simulink model "Progetto_Gruppo21_IZ"  (R2024b)
settings: Solver=FixedStepDiscrete  StartTime=0.0  StopTime=300  FixedStep=0.5  RelTol=1e-3  EnableMultiTasking=on
libraries: stm32f4xxblockslib x6, stm32g4xxblockslib x2, stm32blockslib x2
settings Model: STM32="{\"UARTRead\":{\"ID\":\"Progetto_Gruppo21_IZ:67\"},\"UARTWrite\":{\"ID\":\"Progetto_Gruppo21_IZ:69\"},\"DigitalPortRead\":[{\"ID\":\"Progetto_Gruppo21_IZ:71\"},{\"ID\":\"Progetto_Gruppo21_IZ:72\"},{\"ID\":\"Progetto_Gruppo21_IZ:73\"},{\"ID\":\"Progetto_Gruppo21_IZ:74\"}],\"DigitalPortWrite\":[{\"ID\":\"Progetto_Gruppo21_IZ:75\"},{\"ID\":\"Progetto_Gruppo21_IZ:76\"}],\"PWMOutput\":[{\"ID\":\"Progetto_Gruppo21_IZ:78\"},{\"ID\":\"Progetto_Gruppo21_IZ:80\"}]}"  PacingRate=0.500000  Creator=angel  LastModifiedBy=angel
settings OptimizationCC: DefaultParameterBehavior=Inlined  EnhancedBackFolding=on  PassReuseOutputArgsAs=Individual arguments  ZeroExternalMemoryAtStartup=off  ZeroInternalMemoryAtStartup=off  MaxStackSize=512  OptimizeBlockOrder=speed  DifferentSizesBufferReuse=on  OptimizationCustomize=off  EfficientTunableParamExpr=on
settings DebuggingCC: ParameterTunabilityLossMsg=error
settings HardwareCC: ProdBitPerPointer=32  ProdBitPerSizeT=32  ProdBitPerPtrDiffT=32  ProdLargestAtomicInteger=Long  ProdLargestAtomicFloat=Double  ProdWordSize=32  ProdLongLongMode=on  ProdHWDeviceType=ARM Compatible->ARM Cortex-M
settings RTWCC: Description=Embedded Coder  SystemTargetFile=ert.tlc  HardwareBoard=STM32G4xx Based  TemplateMakefile=ert_default_tmf  Toolchain=GNU Tools for ARM Embedded Processors
settings CodeAppCC: ForceParamTrailComments=on  IgnoreCustomStorageClasses=off  OperatorAnnotations=on  SimulinkDataObjDesc=on  SFDataObjDesc=on  InsertBlockDesc=on
settings ERTTargetCC: TargetLangStandard=C99 (ISO)  CodeReplacementLibrary=ARM Cortex-M  SupportVariableSizeSignals=on  ExtModeTransport=3  ExtModeStaticAlloc=on  ExtModeStaticAllocSize=2048  ExtModeMexFile=ext_xcp  ExtModeIntrfLevel=Level2 - Open

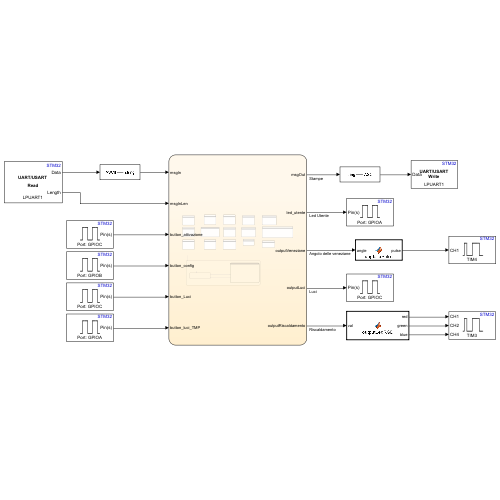
[thumbnail: Simulink's stored preview of the top-level diagram]
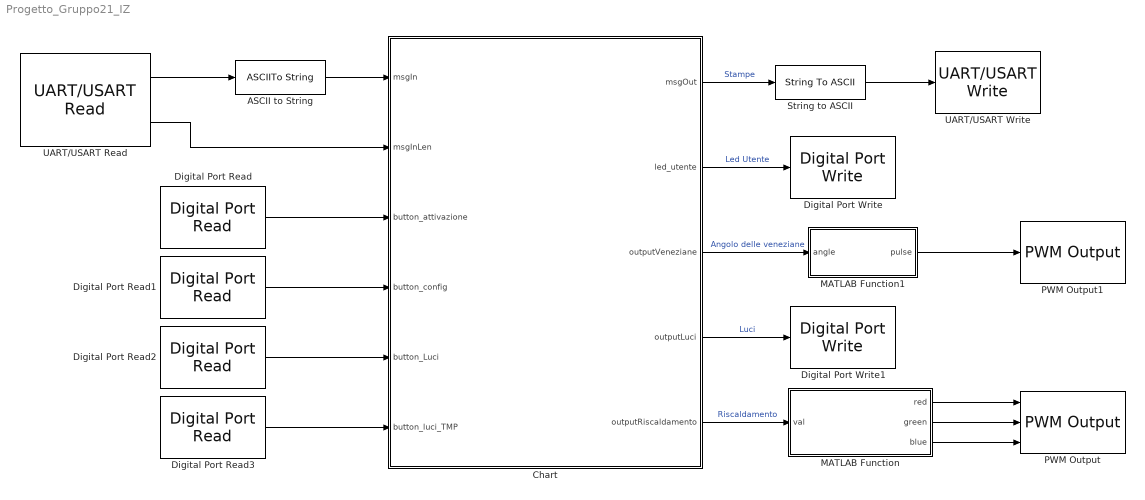
== system Progetto_Gruppo21_IZ ==
  ASCII to String : ASCIIToString
  Chart : Stateflow chart  TreatAsAtomicUnit=on
  Digital Port Read : stm32f4xxblockslib/Digital Port Read  PortName=GPIOC  PinNumber=[13]  ReadOperation=on  IOAsArray=on  SampleTime=-1  EnableSimPort=off  hoistedMaskSrc=ECSoC/ECSimCodegen/Digital Port Read
      settings: LibrarySourceBlock=stm32g4xxblockslib/Digital Port Read
  Digital Port Read1 : stm32f4xxblockslib/Digital Port Read  PortName=GPIOB  PinNumber=[0]  ReadOperation=on  IOAsArray=on  SampleTime=-1  EnableSimPort=off  hoistedMaskSrc=ECSoC/ECSimCodegen/Digital Port Read
      settings: LibrarySourceBlock=stm32g4xxblockslib/Digital Port Read
  Digital Port Read2 : stm32f4xxblockslib/Digital Port Read  PortName=GPIOC  PinNumber=[10]  ReadOperation=on  IOAsArray=on  SampleTime=-1  EnableSimPort=off  hoistedMaskSrc=ECSoC/ECSimCodegen/Digital Port Read
      settings: LibrarySourceBlock=stm32g4xxblockslib/Digital Port Read
  Digital Port Read3 : stm32f4xxblockslib/Digital Port Read  PortName=GPIOA  PinNumber=[15]  ReadOperation=on  IOAsArray=on  SampleTime=-1  EnableSimPort=off  hoistedMaskSrc=ECSoC/ECSimCodegen/Digital Port Read
      settings: LibrarySourceBlock=stm32g4xxblockslib/Digital Port Read
  Digital Port Write : stm32f4xxblockslib/Digital Port Write  PortName=GPIOA  PinNumber=[5]  ReadOperation=off  IOAsArray=on  EnableSimPort=off  hoistedMaskSrc=ECSoC/ECSimCodegen/Digital Port Write
      settings: LibrarySourceBlock=stm32g4xxblockslib/Digital Port Write
  Digital Port Write1 : stm32f4xxblockslib/Digital Port Write  PortName=GPIOC  PinNumber=[2]  ReadOperation=off  IOAsArray=on  EnableSimPort=off  hoistedMaskSrc=ECSoC/ECSimCodegen/Digital Port Write
      settings: LibrarySourceBlock=stm32g4xxblockslib/Digital Port Write
  MATLAB Function : MATLAB Function  TreatAsAtomicUnit=on
  MATLAB Function1 : MATLAB Function  TreatAsAtomicUnit=on
  PWM Output : stm32g4xxblockslib/PWM Output  TimerModule=TIM3  DutycycleUnits=Counts  EnableChannel1=on  EnableChannel2=on  EnableChannel3=off  EnableChannel4=on  EnableChannel5=off  EnableChannel6=off  EnableCounterInput=off  EnableMainOutputInput=off  EnableFrequencyInput=off  SetRCAfterCE=off  OutputDirection=off  OutputMainOutputEnableStatus=off  SampleTime=0.1  EnableSimPort=off  EnableUpdateEvent=off  EnableCaptureCompare1Event=off  EnableCaptureCompare2Event=off  EnableCaptureCompare3Event=off  EnableCaptureCompare4Event=off  EnableTriggerEvent=off  EnableBreakEvent=off  EnableBreakEvent2=off  ProcessorFamily=STM32G4  hoistedMaskSrc=ECSoC/ECSimCodegen/PWM Output
  PWM Output1 : stm32g4xxblockslib/PWM Output  TimerModule=TIM4  DutycycleUnits=Counts  EnableChannel1=on  EnableChannel2=off  EnableChannel3=off  EnableChannel4=off  EnableChannel5=off  EnableChannel6=off  EnableCounterInput=off  EnableMainOutputInput=off  EnableFrequencyInput=off  SetRCAfterCE=off  OutputDirection=off  OutputMainOutputEnableStatus=off  SampleTime=0.1  EnableSimPort=off  EnableUpdateEvent=off  EnableCaptureCompare1Event=off  EnableCaptureCompare2Event=off  EnableCaptureCompare3Event=off  EnableCaptureCompare4Event=off  EnableTriggerEvent=off  EnableBreakEvent=off  EnableBreakEvent2=off  ProcessorFamily=STM32G4  hoistedMaskSrc=ECSoC/ECSimCodegen/PWM Output
  String to ASCII : StringToASCII  OutputVectorSize=127
  UART/USART Read : stm32blockslib/UART//USART Read  UARTModule=LPUART1  DataType=uint8  DataLength=1  BlockingMode=off  BlockingTimeout=0.1  OutputLength=on  OutputStatus=off  SampleTime=-1
      settings: LibrarySourceBlock=stm32g4xxblockslib/UART//USART Read
  UART/USART Write : stm32blockslib/UART//USART Write  UARTModule=LPUART1  LengthOfDataToSend=off  BlockingMode=off  BlockingTimeout=0.1  OutputStatus=off
      settings: LibrarySourceBlock=stm32g4xxblockslib/UART//USART Write
  wires:
  ASCII to String/1 -> Chart/1(msgIn)
  UART/USART Read/1 -> ASCII to String/1
  UART/USART Read/2 -> Chart/2(msgInLen)
  Chart/1(msgOut) -> String to ASCII/1  "Stampe"
  String to ASCII/1 -> UART/USART Write/1
  Digital Port Read/1 -> Chart/3(button_attivazione)
  Digital Port Read1/1 -> Chart/4(button_config)
  Digital Port Read2/1 -> Chart/5(button_Luci)
  Digital Port Read3/1 -> Chart/6(button_luci_TMP)
  Chart/4(outputLuci) -> Digital Port Write1/1  "Luci"
  Chart/2(led_utente) -> Digital Port Write/1  "Led Utente"
  Chart/5(outputRiscaldamento) -> MATLAB Function/1(val)  "Riscaldamento"
  MATLAB Function/1(red) -> PWM Output/1
  MATLAB Function/2(green) -> PWM Output/2
  MATLAB Function/3(blue) -> PWM Output/3
  Chart/3(outputVeneziane) -> MATLAB Function1/1(angle)  "Angolo delle veneziane"
  MATLAB Function1/1(pulse) -> PWM Output1/1

== matlab function Progetto_Gruppo21_IZ/MATLAB Function1 ==
  data: angle input; pulse output
function pulse = angleToPulse(angle)
    pulse = ((angle/180)*2000) + 500;
end

== matlab function Progetto_Gruppo21_IZ/MATLAB Function ==
  data: val input; red output; green output; blue output
function [red,green,blue] = outputLedRGD(val)
    switch val
        case 0
            red = 0;
            green = 0;
            blue = 255;
        case 1
            red = 155;
            green = 0;
            blue = 155;
        case 2
            red = 255;
            green = 90;
            blue = 0;
        case 3
            red = 255;
            green = 20;
            blue = 0;
        case 4
            red = 255;
            green = 0;
            blue = 0;
        otherwise
            red = 0;
            green = 0;
            blue = 0;
end

== stateflow chart Progetto_Gruppo21_IZ/Chart ==
  state Inizializzazione
    state Stato_Attivo
      state Gestione_Pulsanti_Luci [parallel]
        settings: executionOrder=3
        state Stato_di_Attesa
        state Gestore_pulsante_Luci_TMP
          state Caso_luci_accese
            en: luci = 3;
            du:
            if luci ~= 3
            stopTimer = true;
            end
          state Caso_luci_spente
            en: luci = 3;
            outputLuci = ON;
            du:
            if luci ~= 3
            stopTimer = true;
            end
          state Fine_Tempo
            en: luci = 2;
            outputLuci = OFF;
          (default) -> (junction 807) : {stopTimer = false}
          (junction 807) -> Inizializzazione.Stato_Attivo.Gestione_Pulsanti_Luci.Gestore_pulsante_Luci_TMP.Caso_luci_spente [order 2]
          (junction 807) -> Inizializzazione.Stato_Attivo.Gestione_Pulsanti_Luci.Gestore_pulsante_Luci_TMP.Caso_luci_accese [order 1] : [luci == 1]
          Inizializzazione.Stato_Attivo.Gestione_Pulsanti_Luci.Gestore_pulsante_Luci_TMP.Caso_luci_accese -> (junction 801)
          Inizializzazione.Stato_Attivo.Gestione_Pulsanti_Luci.Gestore_pulsante_Luci_TMP.Caso_luci_spente -> (junction 801)
          (junction 801) -> Fine_Tempo [order 2] : after(tempo, sec)
        state Gestore_pulsante_Luci
          state Caso_luci_spente
            en: luci = 1;
            outputLuci = ON;
          state Caso_luci_tmp
            en: luci = 2;
            outputLuci = OFF;
          state Caso_luci_accese
            en: luci = 2;
            outputLuci = OFF;
          (default) -> (junction 798)
          (junction 798) -> Caso_luci_tmp [order 3]
          (junction 798) -> Inizializzazione.Stato_Attivo.Gestione_Pulsanti_Luci.Gestore_pulsante_Luci.Caso_luci_accese [order 1] : [luci == 1]
          (junction 798) -> Inizializzazione.Stato_Attivo.Gestione_Pulsanti_Luci.Gestore_pulsante_Luci.Caso_luci_spente [order 2] : [luci == 2]
          Inizializzazione.Stato_Attivo.Gestione_Pulsanti_Luci.Gestore_pulsante_Luci.Caso_luci_accese -> (junction 799)
          Caso_luci_tmp -> (junction 799)
          Inizializzazione.Stato_Attivo.Gestione_Pulsanti_Luci.Gestore_pulsante_Luci.Caso_luci_spente -> (junction 799)
        (default) -> Stato_di_Attesa
        Stato_di_Attesa -> Gestore_pulsante_Luci [order 1] : [rising(button_Luci) && configurazioneValida]
        Stato_di_Attesa -> Gestore_pulsante_Luci_TMP [order 2] : [rising(button_luci_TMP) && configurazioneValida && valoreTemporizzazione > 0 ]
        (junction 799) -> Stato_di_Attesa
        (junction 801) -> Stato_di_Attesa [order 1] : [stopTimer]
        Fine_Tempo -> Stato_di_Attesa
        Gestore_pulsante_Luci_TMP -> Gestore_pulsante_Luci : [rising(button_Luci)]
      state Gestore_logica [parallel]
        settings: executionOrder=1
        state Stato_Operativo
          state Imposta_parametri [parallel]
            settings: executionOrder=2
            state Imposta_output
              en: outputVeneziane = veneziane;
              outputRiscaldamento = rangeRiscaldamento(riscaldamento);
              state Accendi_luci
                en: outputLuci = ON;
              state Spegni_luci
                en: luci = 2;
                outputLuci = OFF;
              (default) -> (junction 594)
              (junction 594) -> Spegni_luci [order 2]
              (junction 594) -> Accendi_luci [order 1] : [luci == 1]
            (default) -> Imposta_output : {veneziane = valoreVeneziane;
                | riscaldamento = valoreRiscaldamento;
                | luci = modLuci;
                | tempo = valoreTemporizzazione;}
          state Stampa_Stato [parallel]
            settings: executionOrder=1
            state Stampa
              en: msgOut = msgAggiornamentoStato(riscaldamento, veneziane, luci, tempo);
              du: msgOut = "";
            Stampa -> Stampa : after(10, sec)
            (default) -> Stampa : {veneziane = valoreVeneziane;
                | riscaldamento = valoreRiscaldamento;
                | luci = modLuci;
                | tempo = valoreTemporizzazione;}
        state Stato_di_configurazione
          state Uscita_configurazione
            en: msgOut = msgUscita;
            valoreVeneziane = tmpVeneziane;
            valoreRiscaldamento = tmpRiscaldamento;
            valoreTemporizzazione = tmpTemporizzazione;
            modLuci = tmpModLuci;
            du: msgOut = "";
          state Errore_uscita
            en: msgOut = msgErroreUscita;
            du: msgOut = "";
          state Stampa_messaggio_configurazione
            en: msgOut = msgConfigurazione;
            du: msgOut = "";
          state Stato_errore
            en: msgOut = msgErrore;
            du: msgOut = "";
            ex: msg = "";
          state Salva_configurazione
            en: msgOut = msgSalvataggioConfigurazione;
            tmpVeneziane = valoreVeneziane;
            tmpRiscaldamento = valoreRiscaldamento;
            tmpTemporizzazione = valoreTemporizzazione;
            tmpModLuci = modLuci;
            configurazioneValida = true;
            du: msgOut = "";
            ;
          state Regolazione_veneziane
            state Stampa_iniziale
              en: msgOut = msgRegolazioneVeneziane;
              msg = "";
              du: msgOut = "";
            state Buffer_veneziane
              en:msg = msg + msgIn;
              msgOut = msgIn;
              du: msgOut = "";
            state Conferma_valore_veneziane
              en: isValidVeneziane = checkValoreVeneziane(msg);
              msgOut = sprintf('\r\n') + "Controllo valore inserito in corso.";
              du: msgOut = "";
            state Stampa_valore_veneziane
              en: msgOut = sprintf('\r\n') + "Valore valido impostato: " + msg + " gradi.";
              valoreVeneziane = convertitore(msg);
              du: msgOut = "";
              ex: msg = "";
            (default) -> Inizializzazione.Stato_Attivo.Gestore_logica.Stato_di_configurazione.Regolazione_veneziane.Stampa_iniziale
            Inizializzazione.Stato_Attivo.Gestore_logica.Stato_di_configurazione.Regolazione_veneziane.Stampa_iniziale -> Buffer_veneziane : [msgInLen > 0 && msgIn >= '0' && msgIn <= '9']
            Buffer_veneziane -> (junction 313)
            (junction 313) -> Buffer_veneziane [order 2] : [msgInLen > 0 && msgIn >= '0' && msgIn <= '9']
            (junction 313) -> Conferma_valore_veneziane [order 1] : [msgIn == sprintf('\r')]
            Conferma_valore_veneziane -> (junction 317) : after(1, sec)
            (junction 317) -> Stampa_valore_veneziane [order 1] : [isValidVeneziane]
          state Accensione_luci
            state Stampa_iniziale
              en: msgOut = msgAccensioneLuci;
              du: msgOut = "";
            state Luci_temporizzate
              state Stampa_iniziale
                en: msgOut = msgConfigurazioneTemporizzazione;
                du: msgOut = "";
              state Buffer_temporizzazione
                en: msg = msg + msgIn;
                msgOut = msgIn;
                du: msgOut = "";
              state Conferma_valore_temporizzazione
                en: isValidTemporizzazione = checkValoreTemporizzazione(msg);
                msgOut = sprintf('\r\n') + "Controllo valore inserito in corso.";
                du: msgOut = "";
              state Stampa_valore_temporizzazione
                en: msgOut = sprintf('\r\n') + "Valore valido impostato: " + msg + " secondi.";
                valoreTemporizzazione = convertitore(msg);
                du: msgOut = "";
                ex: msg = "";
              (default) -> Inizializzazione.Stato_Attivo.Gestore_logica.Stato_di_configurazione.Accensione_luci.Luci_temporizzate.Stampa_iniziale
              Inizializzazione.Stato_Attivo.Gestore_logica.Stato_di_configurazione.Accensione_luci.Luci_temporizzate.Stampa_iniziale -> Buffer_temporizzazione : [msgInLen > 0 && msgIn >= '0' && msgIn <= '9']
              Buffer_temporizzazione -> (junction 292)
              (junction 292) -> Buffer_temporizzazione [order 2] : [msgInLen > 0 && ((msgIn >= '0' && msgIn <= '9') || msgIn == '.')]
              (junction 292) -> Conferma_valore_temporizzazione [order 1] : [msgIn == sprintf('\r')]
              Conferma_valore_temporizzazione -> (junction 282) : after(1, sec)
              (junction 282) -> Stampa_valore_temporizzazione [order 1] : [isValidTemporizzazione]
            state Luci_accese
              en: modLuci = 1;
              msgOut = sprintf('\r\n') + "Impostazione: Luci accese.";
              du: msgOut = "";
            state Luci_spente
              en: modLuci = 2;
              msgOut = sprintf('\r\n') + "Impostazione: Luci spente.";
              du: msgOut = "";
            (default) -> Inizializzazione.Stato_Attivo.Gestore_logica.Stato_di_configurazione.Accensione_luci.Stampa_iniziale
            (junction 290) -> (junction 698) [order 3]
            (junction 282) -> (junction 698) [order 2]
            Inizializzazione.Stato_Attivo.Gestore_logica.Stato_di_configurazione.Accensione_luci.Stampa_iniziale -> (junction 290) : [msgInLen > 0]
            (junction 290) -> Luci_accese [order 1] : [msgIn == '1']
            (junction 290) -> Luci_spente [order 2] : [msgIn == '2']
            Luci_spente -> Luci_temporizzate : after(1, sec)
            Luci_accese -> Luci_temporizzate : after(1, sec)
          state Configurazione_riscaldamento
            state Stampa_iniziale
              en: msgOut = msgConfigurazioneRiscaldamento;
              msg = "";
              du: msgOut = "";
            state Buffer_riscaldamento
              en: msg = msg + msgIn;
              msgOut = msgIn;
              du: msgOut = "";
            state Conferma_valore_riscaldamento
              en: isValidRiscaldamento = checkValoreRiscaldamento(msg);
              msgOut = sprintf('\r\n') + "Controllo valore inserito in corso.";
              du: msgOut = "";
            state Stampa_valore_riscaldamento
              en: msgOut = sprintf("\r\n") +"Valore valido impostato: " + msg + " gradi.";
              valoreRiscaldamento = convertitore(msg);
              du: msgOut = "";
              ex: msg = "";
            (default) -> Inizializzazione.Stato_Attivo.Gestore_logica.Stato_di_configurazione.Configurazione_riscaldamento.Stampa_iniziale
            Inizializzazione.Stato_Attivo.Gestore_logica.Stato_di_configurazione.Configurazione_riscaldamento.Stampa_iniziale -> Buffer_riscaldamento : [msgInLen > 0 && msgIn >= '0' && msgIn <= '9']
            (junction 271) -> Buffer_riscaldamento [order 2] : [msgInLen > 0 && msgIn >= '0' && msgIn <= '9']
            Buffer_riscaldamento -> (junction 271)
            (junction 271) -> Conferma_valore_riscaldamento [order 1] : [msgIn == sprintf('\r')]
            Conferma_valore_riscaldamento -> (junction 267) : after(1, sec)
            (junction 267) -> Stampa_valore_riscaldamento [order 1] : [isValidRiscaldamento]
          Stampa_valore_temporizzazione -> (junction 689) : after(1, sec)
          (junction 698) -> (junction 687)
          Stato_di_configurazione -> (junction 529) : [rising(button_config)]
          (default) -> Stampa_messaggio_configurazione : {isValidVeneziane = false;
              | isValidRiscaldamento = false;
              | isValidTemporizzazione = false;
              | msg = "";
              | tmpVeneziane = valoreVeneziane;
              | tmpRiscaldamento = valoreRiscaldamento;
              | tmpTemporizzazione = valoreTemporizzazione;
              | tmpModLuci = modLuci;}
          (junction 687) -> Stato_errore
          Errore_uscita -> (junction 689) : after(1, sec)
          (junction 254) -> (junction 687) [order 6]
          (junction 541) -> Errore_uscita [order 1] : [valoreVeneziane == -1 || valoreRiscaldamento == -1 || modLuci == -1 || valoreTemporizzazione == -1]
          (junction 529) -> Errore_uscita [order 1] : [tmpVeneziane == -1 || tmpRiscaldamento == -1 || tmpModLuci == -1 || tmpTemporizzazione == -1]
          (junction 529) -> Uscita_configurazione [order 2]
          (junction 317) -> (junction 687) [order 2]
          Stampa_valore_veneziane -> (junction 689) : after(1, sec)
          Stampa_messaggio_configurazione -> (junction 254) : [msgInLen > 0]
          Stampa_valore_riscaldamento -> (junction 689) : after(1, sec)
          (junction 689) -> Stampa_messaggio_configurazione
          (junction 254) -> (junction 529) [order 5] : [msgIn == '5']
          (junction 267) -> (junction 687) [order 2]
          Stato_errore -> (junction 689) : after(1, sec)
          (junction 254) -> Configurazione_riscaldamento [order 3] : [msgIn == '3']
          (junction 254) -> (junction 541) [order 4] : [msgIn == '4']
          (junction 541) -> Salva_configurazione [order 2]
          (junction 254) -> Regolazione_veneziane [order 1] : [msgIn == '1']
          (junction 254) -> Accensione_luci [order 2] : [msgIn == '2']
        Salva_configurazione -> Stato_Operativo : after(1, sec)
        Uscita_configurazione -> Stato_Operativo : after(1, sec)
        (default) -> (junction 559)
        (junction 559) -> Stato_di_configurazione [order 1] : [~configurazioneValida]
        (junction 559) -> Stato_Operativo [order 2]
        Stato_Operativo -> Stato_di_configurazione : [rising(button_config)]
      state Led_utente [parallel]
        settings: executionOrder=2
        state Accendi_led
          en: led_utente = ON;
        state Spegni_led
          en: led_utente = OFF;
        (default) -> Accendi_led
        Accendi_led -> Spegni_led : after(0.5, sec)
        Spegni_led -> Accendi_led : after(0.5, sec)
    state Stato_Inattivo
      en: msgOut = sprintf("\033[0;0H\033[2J") +"Dispositivo non attivo.";
      led_utente = OFF;
      outputVeneziane = 0;
      outputLuci = OFF;
      outputRiscaldamento = 0;
      du: msgOut = "";
    (default) -> Stato_Inattivo
    Stato_Inattivo -> Stato_Attivo : [rising(button_attivazione)]
    Stato_Attivo -> Stato_Inattivo : [rising(button_attivazione)]{valoreVeneziane = tmpVeneziane;
        |  valoreRiscaldamento = tmpRiscaldamento;
        |  valoreTemporizzazione = tmpTemporizzazione;
        |  modLuci = tmpModLuci;}
  (default) -> Inizializzazione : {valoreVeneziane = -1;
      | valoreRiscaldamento = -1;
      | modLuci = -1;
      | valoreTemporizzazione = -1;
      | configurazioneValida = false;
      | }
  data: outString function_output; outString function_output; outString function_output; outString function_output; outString function_output; outString function_output; val_riscaldamento function_input; val_veneziane function_input; val_luci function_input; val_temporizzazione function_input; outString function_output; outString function_output; outString function_output; outString function_output; str function_input; val function_output; result function_output; str function_input; result function_output; str function_input; result function_output; str function_input; val function_input; outRange function_output; msgOut output string; msgIn input string; msgInLen input; valoreVeneziane local double; valoreRiscaldamento local double; modLuci local double; valoreTemporizzazione local double; msg local string; isValidRiscaldamento local boolean; isValidVeneziane local boolean; isValidTemporizzazione local boolean; tmpVeneziane local double; tmpRiscaldamento local double; tmpTemporizzazione local double; tmpModLuci local double; led_utente output; OFF constant double =0; outputVeneziane output; outputLuci output; button_attivazione input; outputRiscaldamento output; luci local double; riscaldamento local double; tempo local double; veneziane local double; ON constant double =1; button_config input; button_Luci input; button_luci_TMP input; configurazioneValida local boolean; stopTimer local
  function outString = msgConfigurazione:
    | function outString = msgConfigurazione
    | clrscr = sprintf("\033[0;0H\033[2J"); 
    | crlf = sprintf('\r\n');
    | 
    | outString = clrscr + "Configurazione:" + crlf + ...
    |     "1. Regolazione veneziane" + crlf + ...
    |     "2. Accensione luci" + crlf + ...
    |     "3. Configurazione riscaldamento" + crlf + ...
    |     "4. Salva" + crlf + ...;
    |     "5. Esci" + crlf;
    | end
  function outString = msgRegolazioneVeneziane:
    | function outString = msgRegolazioneVeneziane
    | clrscr = sprintf("\033[0;0H\033[2J"); 
    | crlf = sprintf('\r\n');
    | 
    | outString = clrscr + "Regolazione Veneziane." + crlf + ...
    |    "Inserire un valore da 0 a 180." + crlf + ...
    |    "(Risoluzione di 20)" + crlf;
    | end
  function outString = msgAccensioneLuci:
    | function outString = msgAccensioneLuci
    | clrscr = sprintf("\033[0;0H\033[2J"); 
    | crlf = sprintf('\r\n');
    | 
    | outString = clrscr + "Configurazione luci." + crlf + ...
    |     "Inserire:" + crlf + ...
    |     "1. Luci accese." + crlf + ...
    |     "2. Luci spente." + crlf;
    | end
  function outString = msgConfigurazioneRiscaldamento:
    | function outString = msgConfigurazioneRiscaldamento
    | clrscr = sprintf("\033[0;0H\033[2J"); 
    | crlf = sprintf('\r\n');
    | 
    | outString = clrscr + "Configurazione riscaldamento." + crlf + ...
    |     "Inserire un valore compreso tra 16 e 30." + crlf + ...
    |     "(Risoluzione di 1)" + crlf;
    | end
  function outString = msgErroreUscita:
    | function outString = msgErroreUscita
    | clrscr = sprintf("\033[0;0H\033[2J"); 
    | crlf = sprintf('\r\n');
    | 
    | outString = clrscr + "Configurazione valida non presente." + crlf + ...
    |             "Si prega di inserirne una." + crlf;
    | end
  function outString = msgAggiornamentoStato(val_riscaldamento, val_veneziane, val_luci, val_temporizzazione):
    | function outString = msgAggiornamentoStato(val_riscaldamento, val_veneziane, val_luci, val_temporizzazione)
    |     clrscr = sprintf("\033[0;0H\033[2J"); 
    |     crlf = sprintf('\r\n');
    | 
    |     val1 = convertitoreDoubleToString(val_veneziane)
    |     str_veneziane = "Veneziane: " + val1 + " gradi.";
    | 
    |     str_luci = "";
    |     if val_luci == 1 || val_luci == 3
    |         str_luci = "Luci accese.";
    |     else
    |         str_luci = "Luci spente.";
    |     end
    |     
    |     str_tempo = "";
    |     if (val_temporizzazione > 0)
    |        val2 = convertitoreDoubleToString(val_temporizzazione);
    |        str_tempo = "Temporizzazione luci: " + val2 + " secondi.";
    |     else
    |        str_tempo = "Temporizzazione luci non attiva.";
    |     end
    | 
    |     val3 = convertitoreDoubleToString(val_riscaldamento);
    |     str_riscaldamento = "Riscaldamento: " + val3 + " gradi.";
    | 
    |     outString = clrscr + "Stato Operativo:" + crlf + ...
    |        str_veneziane + crlf + ...
    |        str_luci + crlf + ...
    |        str_tempo + crlf + ...
    |        str_riscaldamento + crlf;
    | end
    | 
    | function str = convertitoreDoubleToString(val)
    |    
    |     if val < 0
    |         str = '-';
    |         val = -val;
    |     else
    |         str = '';
    |     end
    | 
    |     parteIntera = floor(val);
    |     parteDecimale = val - parteIntera;
    | 
    |     if parteIntera == 0
    |         str = [str '0'];
    |     else
    |         cifreIntere = '';
    |         while parteIntera > 0
    |             cifra = mod(parteIntera, 10);
    |             cifreIntere = [char(cifra + 48) cifreIntere];
    |             parteIntera = floor(parteIntera / 10);
    |         end
    |         str = [str cifreIntere];
    |     end
    | 
    |     if parteDecimale > 0
    |         str = [str '.'];
    |         for i = 1:2
    |             parteDecimale = parteDecimale * 10;
    |             cifra = floor(parteDecimale);
    |             str = [str char(cifra + 48)];
    |             parteDecimale = parteDecimale - cifra;
    |             if parteDecimale == 0
    |                 break;
    |             end
    |         end
    |     end
    | end
  function outString = msgUscita:
    | function outString = msgUscita
    | clrscr = sprintf("\033[0;0H\033[2J");
    | crlf = sprintf('\r\n');
    | 
    | outString = clrscr + "Uscita in corso." + crlf + ...
    |             "Verranno ripristinate le configurazioni precedenti." + crlf;
    | end
  function outString = msgErrore:
    | function outString = msgErrore
    | clrscr = sprintf("\033[0;0H\033[2J");
    | crlf = sprintf('\r\n');
    | 
    | outString = clrscr + "Valore inserito non valido." + crlf;
    | end
  function outString = msgSalvataggioConfigurazione:
    | function outString = msgSalvataggioConfigurazione
    | clrscr = sprintf("\033[0;0H\033[2J"); 
    | crlf = sprintf('\r\n');
    | 
    | outString = clrscr + "Configurazione salvata con successo." + crlf;
    | end
  function outString = msgConfigurazioneTemporizzazione:
    | function outString = msgConfigurazioneTemporizzazione
    | clrscr = sprintf("\033[0;0H\033[2J"); 
    | crlf = sprintf('\r\n');
    | 
    | outString = clrscr + "Configurazione temporizzazione luci." + crlf + ...
    |     "Inserire un valore compreso tra 5 e 30." + crlf + ...
    |     "Inserire 0 per disattivarla." + crlf;
    | end
  function val = convertitore(str):
    | function val = convertitore(str)
    | 
    |     num = 0;
    |     str = char(str);
    |     isFraction = false;
    |     fractionDivisor = 1;
    | 
    |     for i = 1:length(str)
    |         ch = str(i);
    |         
    |         if ch == ' '
    |             break; 
    |         elseif ch == '.'
    |             if isFraction
    |                 val = -1;
    |                 return;
    |             end
    |             isFraction = true;
    |             continue;
    |         end
    |     
    |         d = double(ch) - 48;
    |         if d < 0 || d > 9
    |             val = -1;
    |             return;
    |         end
    |     
    |         if ~isFraction
    |             num = num * 10 + d;
    |         else
    |             fractionDivisor = fractionDivisor * 10;
    |             num = num + d / fractionDivisor;
    |         end
    |     end
    | 
    |     val = num;
    | 
    | end
  function result = checkValoreRiscaldamento(str):
    | function result = checkValoreRiscaldamento(str)
    | 
    |     num = 0;
    |     str = char(str);
    |     for i = 1:length(str)
    |         if str(i) == ' '
    |             break;
    |         end
    |         d = double(str(i)) - 48;
    |         if d < 0 || d > 9
    |             result = false;
    |             return;
    |         end
    |         num = num * 10 + d;
    |     end
    | 
    |     result = ~isnan(num) && mod(num, 1) == 0 && num >= 16 && num <= 30;
    | end
  function result = checkValoreTemporizzazione(str):
    | function result = checkValoreTemporizzazione(str)
    |   
    |     num = 0;
    |     str = char(str);
    |     isFraction = false;
    |     fractionDivisor = 1;
    | 
    |     for i = 1:length(str)
    |         ch = str(i);
    |         
    |         if ch == ' '
    |             break; 
    |         elseif ch == '.'
    |             if isFraction
    |                 result = false;
    |                 return;
    |             end
    |             isFraction = true;
    |             continue;
    |         end
    |     
    |         d = double(ch) - 48;
    |         if d < 0 || d > 9
    |             result = false;
    |             return;
    |         end
    |     
    |         if ~isFraction
    |             num = num * 10 + d;
    |         else
    |             fractionDivisor = fractionDivisor * 10;
    |             num = num + d / fractionDivisor;
    |         end
    |     end
    | 
    |     result = ~isnan(num) && ((num >= 5 && num <= 30) || num == 0);
    | end
  function result = checkValoreVeneziane(str):
    | function result = checkValoreVeneziane(str)
    |     
    |     num = 0;
    |     str = char(str);
    |     for i = 1:length(str)
    |         if str(i) == ' '
    |             break;
    |         end
    |         d = double(str(i)) - 48;
    |         if d < 0 || d > 9
    |             result = false;
    |             return;
    |         end
    |         num = num * 10 + d;
    |     end
    | 
    |     result = ~isnan(num) && mod(num, 20) == 0 && num >= 0 && num <= 180;
    |     
    | end
  function outRange = rangeRiscaldamento(val):
    | function outRange = rangeRiscaldamento(val)
    | 
    |     if val >= 16 && val <= 18
    |             outRange = 0;
    |     elseif val >= 19 && val <= 21
    |             outRange = 1;
    |     elseif val >= 22 && val <= 24
    |             outRange = 2;
    |     elseif val >= 25 && val <= 27
    |             outRange = 3;
    |     elseif val >= 28 && val <= 30
    |             outRange = 4;
    |     else 
    |         outRange = -1
    |     end
    | 
    | end
